simulink model "MotionControlCompile"  (R2016a)
settings: Solver=ode3  StartTime=0.0  StopTime=inf  FixedStep=0.05  RelTol=1e-3
undefined symbols (not defined in the file or in its folder): C_nuParams, D, D_nuParams, InitialPos, invM, invT, invThrustAloc, K2, K3, K4, Kd, Ki, Kp, MAPP1, MAPP2, MAPP3, Sat1Low, Sat1Up, Sat2Low, Sat2Up, Th1, Th2, Th3, Tr, wni, wniCeta2, wnisquared, X, Y, Z
libraries: robotlib x15, marine_gnc x1
settings Model: Creator=einar  LastModifiedBy=einar
settings DataIOCC: LimitDataPoints=on  ReturnWorkspaceOutputs=on
settings OptimizationCC: OptimizeModelRefInitCode=on  LifeSpan=Inf  MaxStackSize=64
settings DebuggingCC: ReadBeforeWriteMsg=DisableAll  WriteAfterWriteMsg=DisableAll  WriteAfterReadMsg=DisableAll  MultiTaskDSMMsg=none  AllowSymbolicDim=off
settings HardwareCC: ProdBitPerPointer=32  ProdLargestAtomicFloat=None  ProdIntDivRoundTo=Undefined  ProdEndianess=Unspecified  ProdWordSize=32  ProdHWDeviceType=Generic->Unspecified (assume 32-bit Generic)
settings ModelReferenceCC: UpdateModelReferenceTargets=IfOutOfDate  PropagateSignalLabelsOutOfModel=off
settings SFSimCC: SFSimEcho=off
settings RTWCC: SystemTargetFile=ert.tlc  HardwareBoard=Robot Operating System (ROS)  TemplateMakefile=ert_default_tmf  Toolchain=Catkin  TargetLang=C++
settings CodeAppCC: IgnoreCustomStorageClasses=off
settings ERTTargetCC: SupportContinuousTime=on  ConvertIfToSwitch=off  SuppressUnreachableDefaultCases=off

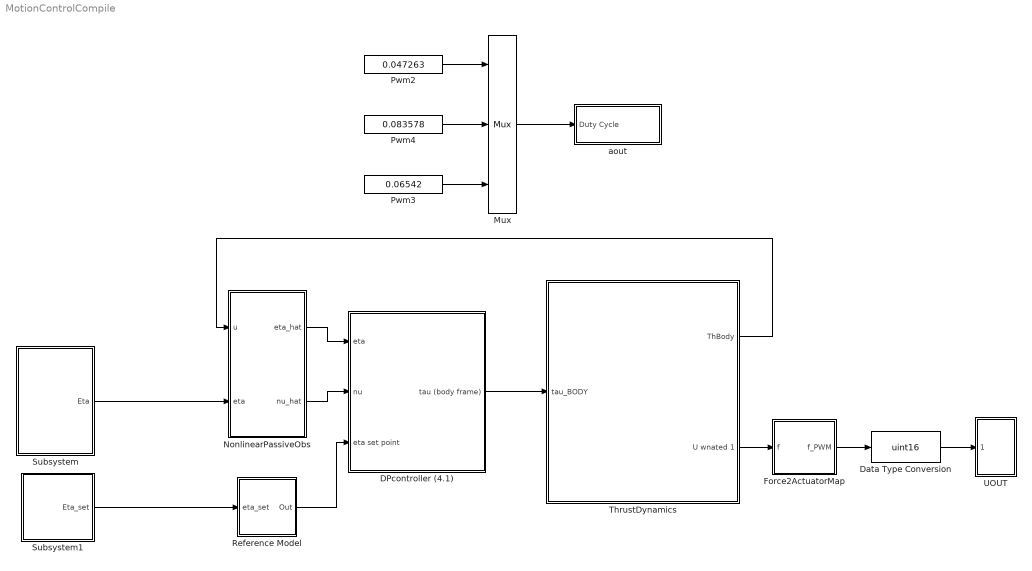
== system MotionControlCompile ==
  DPcontroller (4.1) : Subsystem
  Data Type Conversion : DataTypeConversion  OutDataTypeStr=uint16
  Force2ActuatorMap : Subsystem
  Mux : Mux  Inputs=3
  NonlinearPassiveObs : Subsystem
  Pwm2 : Constant  Value=0.047263
  Pwm3 : Constant  Value=0.06542
  Pwm4 : Constant  Value=0.083578
  Reference Model : Subsystem
  Subsystem : Subsystem
  Subsystem1 : Subsystem
  ThrustDynamics : Subsystem
  UOUT : Subsystem
  aout : Subsystem
  wires:
  NonlinearPassiveObs/2(nu_hat) -> DPcontroller (4.1)/2(nu)
  Reference Model/1(Out) -> DPcontroller (4.1)/3(eta set point)
  NonlinearPassiveObs/1(eta_hat) -> DPcontroller (4.1)/1(eta)
  ThrustDynamics/2(U wnated 1) -> Force2ActuatorMap/1(f)
  Data Type Conversion/1 -> UOUT/1(f_PWM)
  Force2ActuatorMap/1(f_PWM) -> Data Type Conversion/1
  DPcontroller (4.1)/1(tau (body frame)) -> ThrustDynamics/1(tau_BODY)
  ThrustDynamics/1("ThBody ") -> NonlinearPassiveObs/1(u)
  Pwm4/1 -> Mux/2
  Pwm2/1 -> Mux/1
  Pwm3/1 -> Mux/3
  Mux/1 -> aout/1(Duty Cycle)
  Subsystem1/1(Eta_set) -> Reference Model/1(eta_set)
  Subsystem/1(Eta) -> NonlinearPassiveObs/2(eta)

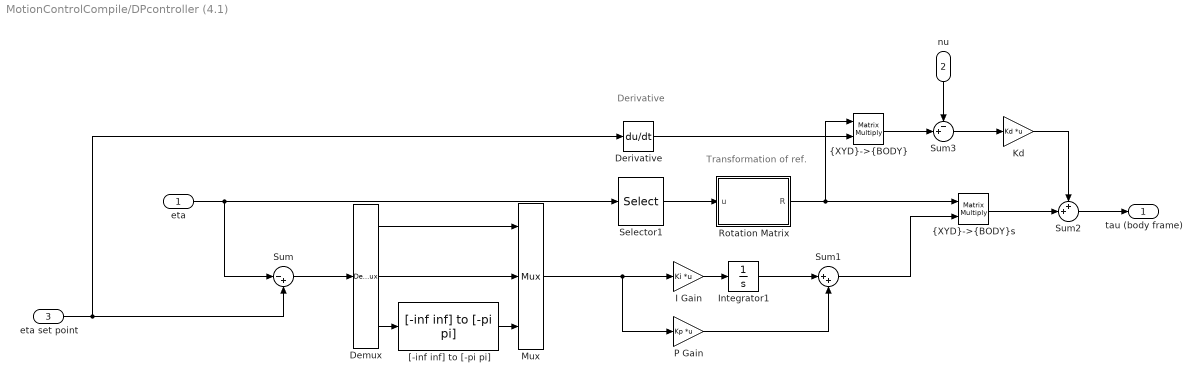
== system MotionControlCompile/DPcontroller (4.1) ==
  note: Transformation of ref.
  note: Derivative
  eta : Inport
  nu : Inport  Port=2
  eta set point : Inport  Port=3
  Demux : Demux  Outputs=3
  Derivative : Derivative
  I Gain : Gain  Gain=Ki  Multiplication=Matrix(K*u)
  Integrator1 : Integrator  InitialCondition=[0;0;0]  LimitOutput=on  UpperSaturationLimit=[1;1;1]  LowerSaturationLimit=[-1;-1;-1]
  Kd : Gain  Gain=Kd  Multiplication=Matrix(K*u)
  Mux : Mux  Inputs=3
  P Gain : Gain  Gain=Kp  Multiplication=Matrix(K*u)
  Rotation Matrix : MATLAB Function  TreatAsAtomicUnit=on
  Selector1 : Selector  InputPortWidth=3  IndexOptions=Index vector (dialog)  Indices=[3]  OutputSizes=1
  Sum : Sum  Inputs=|-+
  Sum1 : Sum  Inputs=|++
  Sum2 : Sum  Inputs=++|
  Sum3 : Sum  Inputs=-+|
  "[-inf inf] to [-pi pi]" : marine_gnc/Utilities/Math Operations/[-inf inf] to [-pi pi]
  "{XYD}->{BODY}" : Product  Multiplication=Matrix(*)
  "{XYD}->{BODY}s" : Product  Multiplication=Matrix(*)
  tau (body frame) : Outport
  wires:
  eta/1 -> Selector1/1, Sum/1
  Selector1/1 -> Rotation Matrix/1(u)
  Rotation Matrix/1(R) -> "{XYD}->{BODY}"/1, "{XYD}->{BODY}s"/1
  Sum2/1 -> tau (body frame)/1
  I Gain/1 -> Integrator1/1
  P Gain/1 -> Sum1/2
  Sum1/1 -> "{XYD}->{BODY}s"/2
  Derivative/1 -> "{XYD}->{BODY}"/2
  "{XYD}->{BODY}s"/1 -> Sum2/2
  nu/1 -> Sum3/1
  "{XYD}->{BODY}"/1 -> Sum3/2
  Sum3/1 -> Kd/1
  Kd/1 -> Sum2/1
  eta set point/1 -> Sum/2, Derivative/1
  Integrator1/1 -> Sum1/1
  Demux/1 -> Mux/1
  Demux/3 -> "[-inf inf] to [-pi pi]"/1
  "[-inf inf] to [-pi pi]"/1 -> Mux/3
  Demux/2 -> Mux/2
  Sum/1 -> Demux/1
  Mux/1 -> P Gain/1, I Gain/1

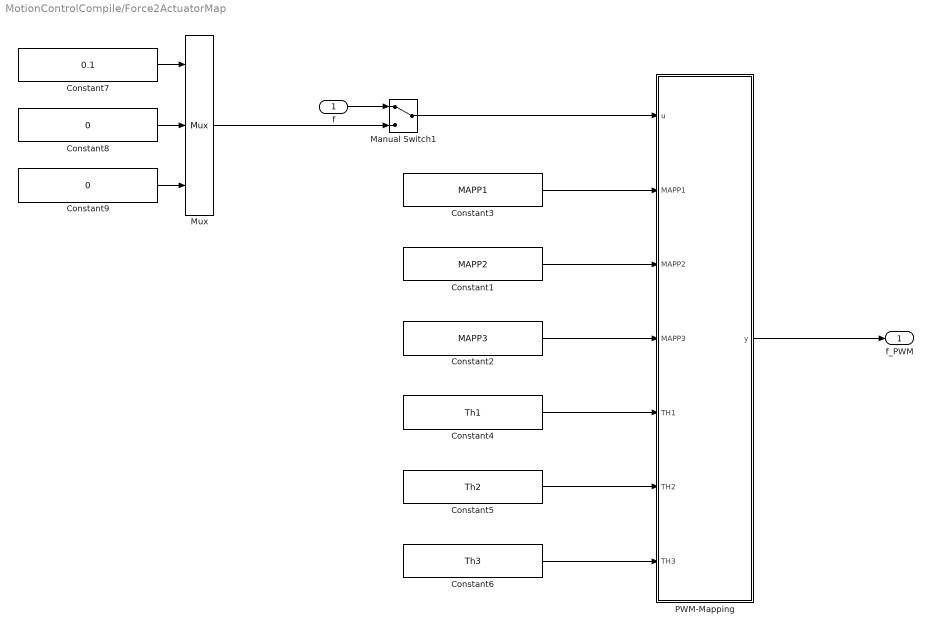
== system MotionControlCompile/Force2ActuatorMap ==
  f : Inport
  Constant1 : Constant  Value=MAPP2
  Constant2 : Constant  Value=MAPP3
  Constant3 : Constant  Value=MAPP1
  Constant4 : Constant  Value=Th1
  Constant5 : Constant  Value=Th2
  Constant6 : Constant  Value=Th3
  Constant7 : Constant  Value=0.1
  Constant8 : Constant  Value=0
  Constant9 : Constant  Value=0
  Manual Switch1 : ManualSwitch
  Mux : Mux  Inputs=3
  PWM-Mapping : MATLAB Function  TreatAsAtomicUnit=on
  f_PWM : Outport
  wires:
  Manual Switch1/1 -> PWM-Mapping/1(u)
  Constant4/1 -> PWM-Mapping/5(TH1)
  Constant6/1 -> PWM-Mapping/7(TH3)
  Constant5/1 -> PWM-Mapping/6(TH2)
  Constant3/1 -> PWM-Mapping/2(MAPP1)
  Constant1/1 -> PWM-Mapping/3(MAPP2)
  Constant2/1 -> PWM-Mapping/4(MAPP3)
  PWM-Mapping/1(y) -> f_PWM/1
  f/1 -> Manual Switch1/1
  Constant7/1 -> Mux/1
  Constant8/1 -> Mux/2
  Mux/1 -> Manual Switch1/2
  Constant9/1 -> Mux/3

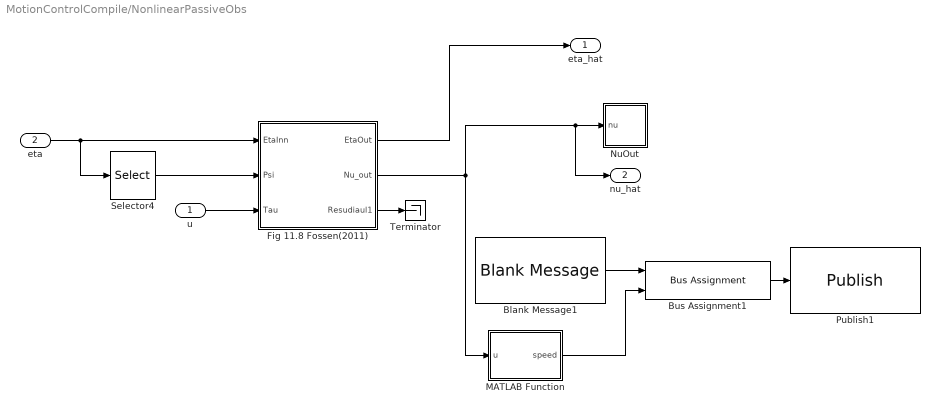
== system MotionControlCompile/NonlinearPassiveObs ==
  u : Inport
  eta : Inport  Port=2
  Blank Message1 : robotlib/Blank Message  SourceLibraryInfo=This block requires Robotics System Toolbox  messageType=std_msgs/Float64  SampleTime=inf
  Bus Assignment1 : BusAssignment  AssignedSignals=Data
  Fig 11.8 Fossen(2011) : Subsystem
  MATLAB Function : MATLAB Function  TreatAsAtomicUnit=on
  NuOut : Subsystem
  Publish1 : robotlib/Publish  SourceLibraryInfo=This block requires Robotics System Toolbox  topicSource=Specify your own  topic=/VesselSpeed  messageType=std_msgs/Float64  messageQueueLength=1
  Selector4 : Selector  InputPortWidth=3  IndexOptions=Index vector (dialog)  Indices=3  OutputSizes=1
  Terminator : Terminator
  eta_hat : Outport
  nu_hat : Outport  Port=2
  wires:
  Fig 11.8 Fossen(2011)/3("Resudiaul1 ") -> Terminator/1
  eta/1 -> Fig 11.8 Fossen(2011)/1(EtaInn), Selector4/1
  Selector4/1 -> Fig 11.8 Fossen(2011)/2(Psi)
  u/1 -> Fig 11.8 Fossen(2011)/3("Tau ")
  Fig 11.8 Fossen(2011)/1("EtaOut ") -> eta_hat/1
  Bus Assignment1/1 -> Publish1/1
  Blank Message1/1 -> Bus Assignment1/1
  Fig 11.8 Fossen(2011)/2("Nu_out ") -> nu_hat/1, NuOut/1("nu "), MATLAB Function/1(u)
  MATLAB Function/1(speed) -> Bus Assignment1/2

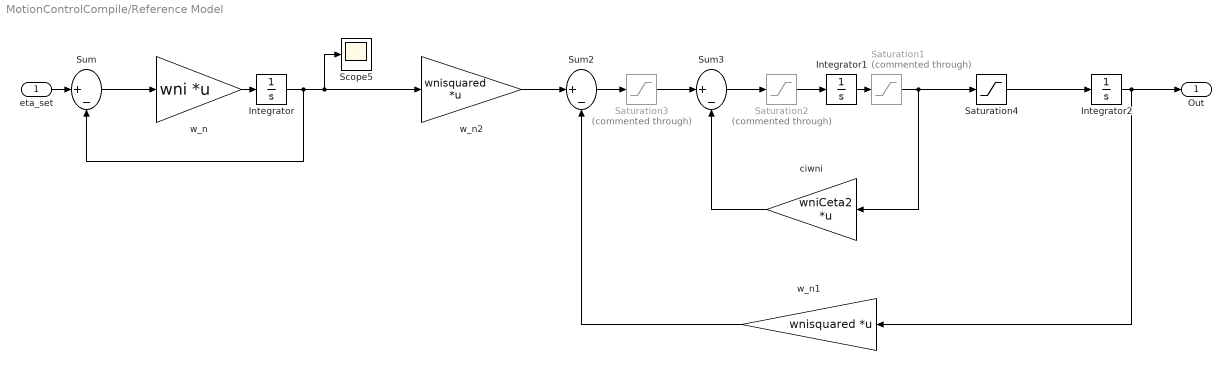
== system MotionControlCompile/Reference Model ==
  eta_set : Inport
  Integrator : Integrator  InitialCondition=[0;0;0]
  Integrator1 : Integrator  InitialCondition=[0 ;0; 0]
  Integrator2 : Integrator  InitialCondition=[0;0;0]
  Saturation1 : Saturate  Commented=through  UpperLimit=Sat2Up  LowerLimit=Sat2Low
  Saturation2 : Saturate  Commented=through  UpperLimit=Sat1Up  LowerLimit=Sat1Low
  Saturation3 : Saturate  Commented=through  UpperLimit=Sat1Up  LowerLimit=Sat1Low
  Saturation4 : Saturate  UpperLimit=Sat2Up  LowerLimit=Sat2Low
  Scope5 : Scope
  Sum : Sum  Inputs=|+-
  Sum2 : Sum  Inputs=|+-
  Sum3 : Sum  Inputs=|+-
  ciwni : Gain  Gain=wniCeta2  Multiplication=Matrix(K*u)
  w_n : Gain  Gain=wni  Multiplication=Matrix(K*u)
  w_n1 : Gain  Gain=wnisquared  Multiplication=Matrix(K*u)
  w_n2 : Gain  Gain=wnisquared  Multiplication=Matrix(K*u)
  Out : Outport
  wires:
  w_n/1 -> Integrator/1
  w_n2/1 -> Sum2/1
  Integrator/1 -> Scope5/1, w_n2/1, Sum/2
  Integrator2/1 -> Out/1, w_n1/1
  ciwni/1 -> Sum3/2
  Saturation1/1 -> ciwni/1, Saturation4/1
  Saturation2/1 -> Integrator1/1
  Sum2/1 -> Saturation3/1
  Sum3/1 -> Saturation2/1
  Sum/1 -> w_n/1
  eta_set/1 -> Sum/1
  Integrator1/1 -> Saturation1/1
  w_n1/1 -> Sum2/2
  Saturation3/1 -> Sum3/1
  Saturation4/1 -> Integrator2/1

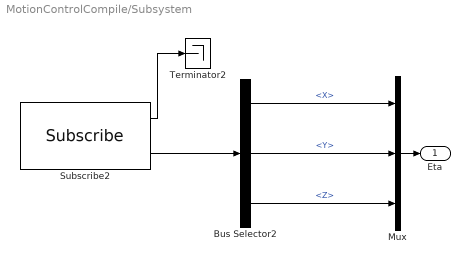
== system MotionControlCompile/Subsystem ==
  Bus Selector2 : BusSelector  OutputSignals=X,Y,Z
  Mux : Mux  Inputs=3
  Subscribe2 : robotlib/Subscribe  SourceLibraryInfo=This block requires Robotics System Toolbox  topicSource=Specify your own  topic=/Position  messageType=geometry_msgs/Vector3  sampleTime=-1  messageQueueLength=1
  Terminator2 : Terminator
  Eta : Outport
  wires:
  Bus Selector2/1 -> Mux/1  "<X>"
  Subscribe2/2 -> Bus Selector2/1
  Mux/1 -> Eta/1
  Subscribe2/1 -> Terminator2/1
  Bus Selector2/3 -> Mux/3  "<Z>"
  Bus Selector2/2 -> Mux/2  "<Y>"

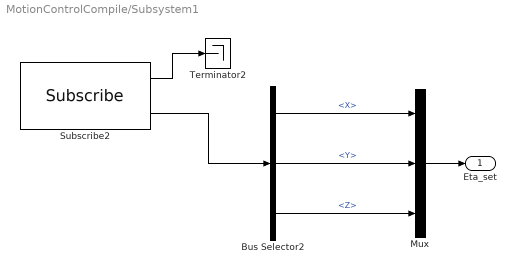
== system MotionControlCompile/Subsystem1 ==
  Bus Selector2 : BusSelector  OutputSignals=X,Y,Z
  Mux : Mux  Inputs=3
  Subscribe2 : robotlib/Subscribe  SourceLibraryInfo=This block requires Robotics System Toolbox  topicSource=Specify your own  topic=/SetPoint  messageType=geometry_msgs/Vector3  sampleTime=-1  messageQueueLength=1
  Terminator2 : Terminator
  Eta_set : Outport
  wires:
  Subscribe2/2 -> Bus Selector2/1
  Mux/1 -> Eta_set/1
  Subscribe2/1 -> Terminator2/1
  Bus Selector2/1 -> Mux/1  "<X>"
  Bus Selector2/2 -> Mux/2  "<Y>"
  Bus Selector2/3 -> Mux/3  "<Z>"

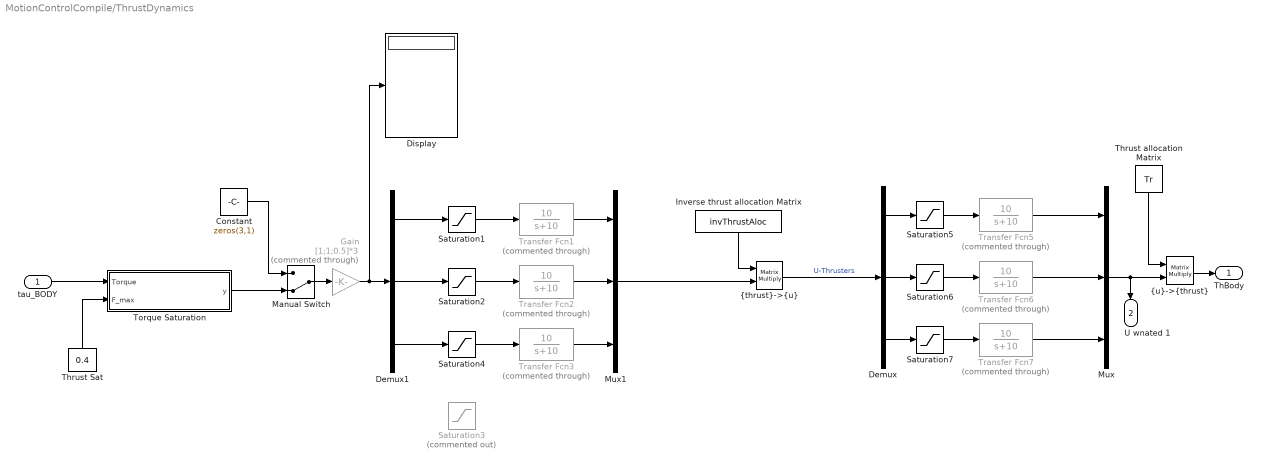
== system MotionControlCompile/ThrustDynamics ==
  tau_BODY : Inport
  Constant : Constant  Value=zeros(3,1)
  Demux : Demux  Outputs=3
  Demux1 : Demux  Outputs=3
  Display : Display
  Gain : Gain  Commented=through  Gain=[1;1;0.5]*3
  Inverse thrust allocation Matrix : Constant  Value=invThrustAloc
  Manual Switch : ManualSwitch  CurrentSetting=0
  Mux : Mux  Inputs=3
  Mux1 : Mux  Inputs=3
  Saturation1 : Saturate  UpperLimit=1  LowerLimit=-1  ZeroCross=off
  Saturation2 : Saturate  UpperLimit=1  LowerLimit=-1  ZeroCross=off
  Saturation3 : Saturate  Commented=on  UpperLimit=0.05  LowerLimit=-0.05  ZeroCross=off
  Saturation4 : Saturate  UpperLimit=1  LowerLimit=-1  ZeroCross=off
  Saturation5 : Saturate  UpperLimit=4  LowerLimit=-4  ZeroCross=off
  Saturation6 : Saturate  UpperLimit=4  LowerLimit=-4  ZeroCross=off
  Saturation7 : Saturate  UpperLimit=4  LowerLimit=-4  ZeroCross=off
  Thrust Sat : Constant  Value=0.4
  Thrust allocation Matrix : Constant  Value=Tr
  Torque Saturation : MATLAB Function  TreatAsAtomicUnit=on
  Transfer Fcn{1..3,5..7} (6 alike) : TransferFcn  Commented=through  Numerator=[10]  Denominator=[1 10]
  "{thrust}->{u}" : Product  Multiplication=Matrix(*)
  "{u}->{thrust}" : Product  Multiplication=Matrix(*)
  "ThBody " : Outport
  U wnated 1 : Outport  Port=2
  wires:
  Demux/1 -> Saturation5/1
  Demux/2 -> Saturation6/1
  Demux/3 -> Saturation7/1
  "{u}->{thrust}"/1 -> "ThBody "/1
  Thrust allocation Matrix/1 -> "{u}->{thrust}"/1
  Mux/1 -> "{u}->{thrust}"/2, U wnated 1/1
  "{thrust}->{u}"/1 -> Demux/1  "U-Thrusters"
  Inverse thrust allocation Matrix/1 -> "{thrust}->{u}"/1
  Saturation7/1 -> Transfer Fcn7/1
  Saturation6/1 -> Transfer Fcn6/1
  Saturation5/1 -> Transfer Fcn5/1
  Transfer Fcn5/1 -> Mux/1
  Transfer Fcn7/1 -> Mux/3
  Transfer Fcn6/1 -> Mux/2
  tau_BODY/1 -> Torque Saturation/1(Torque)
  Demux1/1 -> Saturation1/1
  Demux1/2 -> Saturation2/1
  Demux1/3 -> Saturation4/1
  Saturation4/1 -> Transfer Fcn3/1
  Saturation2/1 -> Transfer Fcn2/1
  Saturation1/1 -> Transfer Fcn1/1
  Transfer Fcn1/1 -> Mux1/1
  Transfer Fcn3/1 -> Mux1/3
  Transfer Fcn2/1 -> Mux1/2
  Gain/1 -> Display/1, Demux1/1
  Mux1/1 -> "{thrust}->{u}"/2
  Thrust Sat/1 -> Torque Saturation/2(F_max)
  Torque Saturation/1(y) -> Manual Switch/2
  Manual Switch/1 -> Gain/1
  Constant/1 -> Manual Switch/1

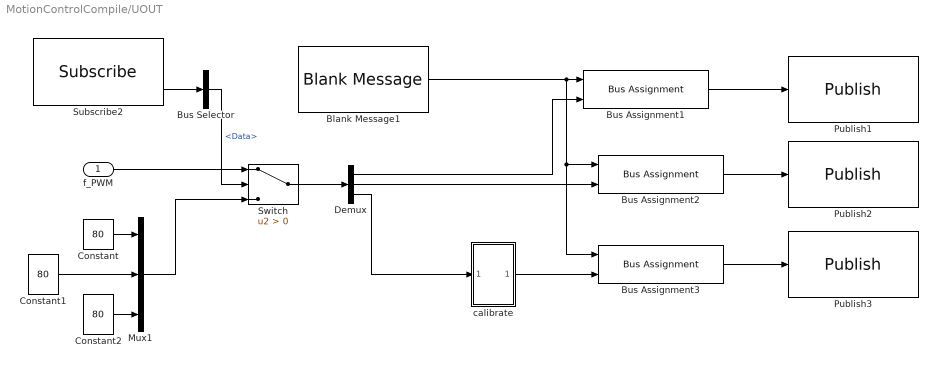
== system MotionControlCompile/UOUT ==
  f_PWM : Inport
  Blank Message1 : robotlib/Blank Message  SourceLibraryInfo=This block requires Robotics System Toolbox  messageType=std_msgs/UInt16  SampleTime=inf
  Bus Assignment1 : BusAssignment  AssignedSignals=Data
  Bus Assignment2 : BusAssignment  AssignedSignals=Data
  Bus Assignment3 : BusAssignment  AssignedSignals=Data
  Bus Selector : BusSelector  OutputSignals=Data
  Constant : Constant  Value=80  OutDataTypeStr=uint16
  Constant1 : Constant  Value=80  OutDataTypeStr=uint16
  Constant2 : Constant  Value=80  OutDataTypeStr=uint16
  Demux : Demux  Outputs=3
  Mux1 : Mux  Inputs=3
  Publish1 : robotlib/Publish  SourceLibraryInfo=This block requires Robotics System Toolbox  topicSource=Specify your own  topic=/Thrust1  messageType=std_msgs/UInt16  messageQueueLength=1
  Publish2 : robotlib/Publish  SourceLibraryInfo=This block requires Robotics System Toolbox  topicSource=Specify your own  topic=/Thrust2  messageType=std_msgs/UInt16  messageQueueLength=1
  Publish3 : robotlib/Publish  SourceLibraryInfo=This block requires Robotics System Toolbox  topicSource=Specify your own  topic=/Thrust3  messageType=std_msgs/UInt16  messageQueueLength=1
  Subscribe2 : robotlib/Subscribe  SourceLibraryInfo=This block requires Robotics System Toolbox  topicSource=Specify your own  topic=/Motor_on_off  messageType=std_msgs/Bool  sampleTime=-1  messageQueueLength=1
  Switch : Switch  Criteria=u2 > Threshold
  calibrate : Subsystem
  wires:
  Bus Assignment3/1 -> Publish3/1
  Demux/2 -> Bus Assignment2/2
  Bus Assignment1/1 -> Publish1/1
  Blank Message1/1 -> Bus Assignment3/1, Bus Assignment2/1, Bus Assignment1/1
  f_PWM/1 -> Switch/1
  Demux/1 -> Bus Assignment1/2
  Bus Assignment2/1 -> Publish2/1
  Switch/1 -> Demux/1
  Mux1/1 -> Switch/3
  Constant/1 -> Mux1/1
  Constant1/1 -> Mux1/2
  Constant2/1 -> Mux1/3
  Subscribe2/2 -> Bus Selector/1
  Bus Selector/1 -> Switch/2  "<Data>"
  Demux/3 -> calibrate/1(In1)
  calibrate/1(Out1) -> Bus Assignment3/2

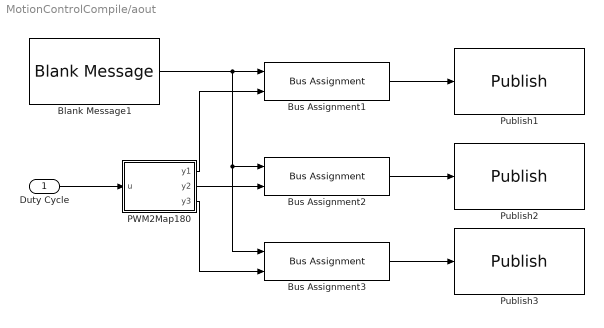
== system MotionControlCompile/aout ==
  Duty Cycle : Inport
  Blank Message1 : robotlib/Blank Message  SourceLibraryInfo=This block requires Robotics System Toolbox  messageType=std_msgs/UInt16  SampleTime=inf
  Bus Assignment1 : BusAssignment  AssignedSignals=Data
  Bus Assignment2 : BusAssignment  AssignedSignals=Data
  Bus Assignment3 : BusAssignment  AssignedSignals=Data
  PWM2Map180 : MATLAB Function  TreatAsAtomicUnit=on
  Publish1 : robotlib/Publish  SourceLibraryInfo=This block requires Robotics System Toolbox  topicSource=Specify your own  topic=/a1  messageType=std_msgs/UInt16  messageQueueLength=1
  Publish2 : robotlib/Publish  SourceLibraryInfo=This block requires Robotics System Toolbox  topicSource=Specify your own  topic=/a2  messageType=std_msgs/UInt16  messageQueueLength=1
  Publish3 : robotlib/Publish  SourceLibraryInfo=This block requires Robotics System Toolbox  topicSource=Specify your own  topic=/a3  messageType=std_msgs/UInt16  messageQueueLength=1
  wires:
  Bus Assignment2/1 -> Publish2/1
  PWM2Map180/1(y1) -> Bus Assignment1/2
  PWM2Map180/3(y3) -> Bus Assignment3/2
  Duty Cycle/1 -> PWM2Map180/1(u)
  Blank Message1/1 -> Bus Assignment1/1, Bus Assignment2/1, Bus Assignment3/1
  Bus Assignment1/1 -> Publish1/1
  PWM2Map180/2(y2) -> Bus Assignment2/2
  Bus Assignment3/1 -> Publish3/1

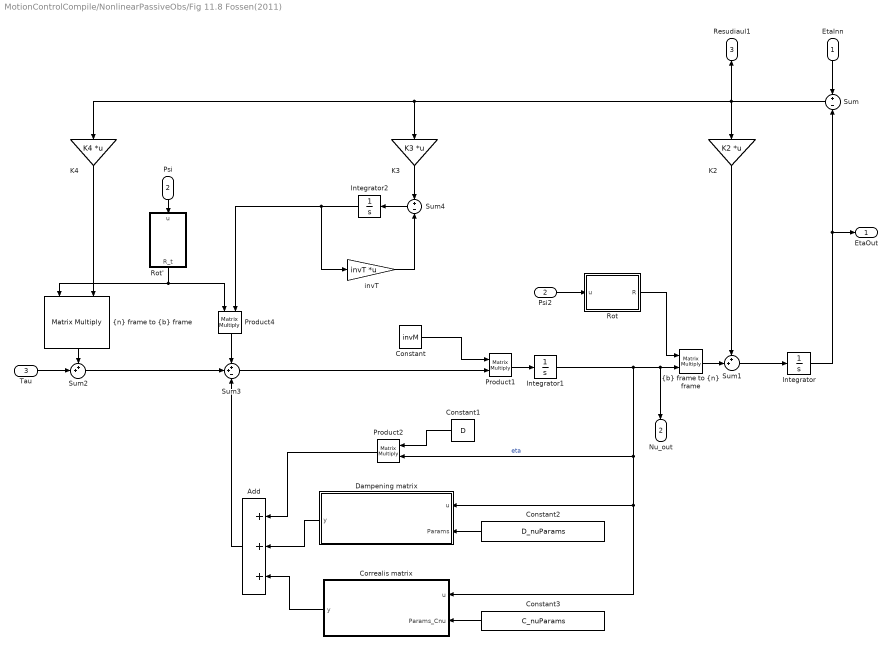
== system MotionControlCompile/NonlinearPassiveObs/Fig 11.8 Fossen(2011) ==
  EtaInn : Inport
  Psi : Inport  Port=2
  "Tau " : Inport  Port=3
  Add : Sum  Inputs=+++
  Constant : Constant  Value=invM
  Constant1 : Constant  Value=D
  Constant2 : Constant  Value=D_nuParams
  Constant3 : Constant  Value=C_nuParams
  Correalis matrix : MATLAB Function  TreatAsAtomicUnit=on
  Dampening matrix : MATLAB Function  TreatAsAtomicUnit=on
  Integrator : Integrator  InitialCondition=InitialPos
  Integrator1 : Integrator
  Integrator2 : Integrator  InitialCondition=[0;0;0]
  K2 : Gain  Gain=K2  Multiplication=Matrix(K*u)
  K3 : Gain  Gain=K3  Multiplication=Matrix(K*u)
  K4 : Gain  Gain=K4  Multiplication=Matrix(K*u)
  Product1 : Product  Multiplication=Matrix(*)
  Product2 : Product  Multiplication=Matrix(*)
  Product4 : Product  Multiplication=Matrix(*)
  Psi2 : InportShadow  Port=2
  Rot : MATLAB Function  TreatAsAtomicUnit=on
  Rot' : MATLAB Function  TreatAsAtomicUnit=on
  Sum : Sum  Inputs=+|-
  Sum1 : Sum  Inputs=++|
  Sum2 : Sum  Inputs=++|
  Sum3 : Sum  Inputs=++-
  Sum4 : Sum  Inputs=+|-
  invT : Gain  Gain=invT  Multiplication=Matrix(K*u)
  "{b} frame to {n} frame" : Product  Multiplication=Matrix(*)
  "{n} frame to {b} frame" : Product  Multiplication=Matrix(*)
  "EtaOut " : Outport
  "Nu_out " : Outport  Port=2
  "Resudiaul1 " : Outport  Port=3
  wires:
  Add/1 -> Sum3/3
  Correalis matrix/1(y) -> Add/3
  Dampening matrix/1(y) -> Add/2
  Product2/1 -> Add/1
  Integrator1/1 -> "{b} frame to {n} frame"/2, "Nu_out "/1, Product2/2, Dampening matrix/1(u), Correalis matrix/1(u)  "eta"
  Constant3/1 -> Correalis matrix/2(Params_Cnu)
  Constant2/1 -> Dampening matrix/2(Params)
  K4/1 -> "{n} frame to {b} frame"/2
  EtaInn/1 -> Sum/1
  Sum/1 -> "Resudiaul1 "/1, K4/1, K3/1, K2/1
  K2/1 -> Sum1/1
  Sum1/1 -> Integrator/1
  Integrator/1 -> Sum/2, "EtaOut "/1
  Psi/1 -> Rot'/1(u)
  "{n} frame to {b} frame"/1 -> Sum2/1
  "Tau "/1 -> Sum2/2
  Constant/1 -> Product1/1
  Product1/1 -> Integrator1/1
  Constant1/1 -> Product2/1
  Sum2/1 -> Sum3/2
  Sum3/1 -> Product1/2
  Psi2/1 -> Rot/1(u)
  Rot/1(R) -> "{b} frame to {n} frame"/1
  Rot'/1(R_t) -> "{n} frame to {b} frame"/1, Product4/1
  "{b} frame to {n} frame"/1 -> Sum1/2
  K3/1 -> Sum4/1
  Sum4/1 -> Integrator2/1
  Integrator2/1 -> Product4/2, invT/1
  invT/1 -> Sum4/2
  Product4/1 -> Sum3/1

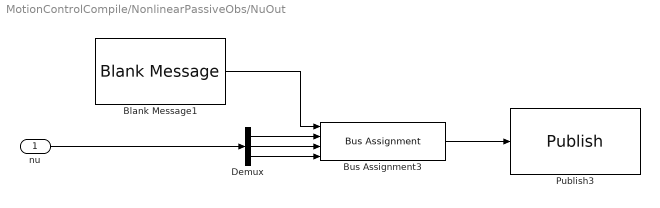
== system MotionControlCompile/NonlinearPassiveObs/NuOut ==
  "nu " : Inport
  Blank Message1 : robotlib/Blank Message  SourceLibraryInfo=This block requires Robotics System Toolbox  messageType=geometry_msgs/Vector3  SampleTime=inf
  Bus Assignment3 : BusAssignment  AssignedSignals=X,Y,Z
  Demux : Demux  Outputs=3
  Publish3 : robotlib/Publish  SourceLibraryInfo=This block requires Robotics System Toolbox  topicSource=Specify your own  topic=/nu  messageType=geometry_msgs/Vector3  messageQueueLength=1
  wires:
  Bus Assignment3/1 -> Publish3/1
  Blank Message1/1 -> Bus Assignment3/1
  "nu "/1 -> Demux/1
  Demux/1 -> Bus Assignment3/2
  Demux/2 -> Bus Assignment3/3
  Demux/3 -> Bus Assignment3/4

== system MotionControlCompile/UOUT/calibrate ==
  In1 : Inport
  Calibrate : MATLAB Function  TreatAsAtomicUnit=on
  Data Type Conversion : DataTypeConversion  OutDataTypeStr=int16
  Data Type Conversion1 : DataTypeConversion  OutDataTypeStr=uint16
  Out1 : Outport
  wires:
  Data Type Conversion/1 -> Calibrate/1(u)
  Calibrate/1(y) -> Data Type Conversion1/1
  Data Type Conversion1/1 -> Out1/1
  In1/1 -> Data Type Conversion/1

== matlab function MotionControlCompile/DPcontroller (4.1)/Rotation Matrix ==
  data: u input; R output
function R = fcn(u)
RotPhi=[cos(u) -sin(u) 0;sin(u) cos(u) 0 ;0 0 1];
R = RotPhi';
%R=[RotPhi(1:2,:);[0 0 0;0 0 0;0 0 0];RotPhi(3,:)]
end

== matlab function MotionControlCompile/NonlinearPassiveObs/Fig 11.8 Fossen(2011)/Correalis matrix ==
  data: u input; y output; Params_Cnu input
function y = fcn(u,Params_Cnu)
%#codegen
C=[0 Params_Cnu(2,1)*u(3) 0;-Params_Cnu(1,2)*u(3) 0 0;0 0 0];
y=C*u;

== matlab function MotionControlCompile/NonlinearPassiveObs/Fig 11.8 Fossen(2011)/Dampening matrix ==
  data: u input; y output; Params input
function y = fcn(u,Params)
%#codegen
Dnu=[Params(1,1)*abs(u(1)) 0 0;0 Params(2,2)*abs(u(2)) 0;0 0 0];
y=Dnu*u;

== matlab function MotionControlCompile/Force2ActuatorMap/PWM-Mapping ==
  data: u input; y output; MAPP1 input; MAPP2 input; MAPP3 input; TH1 input; TH2 input; TH3 input
function y = fcn(u,MAPP1,MAPP2,MAPP3,TH1,TH2,TH3)
y=[0 ;0;0]
u(3)=-u(3);
MAPP3=-MAPP1;
TH3=TH1

if u(1)>max(MAPP1)
    u(1)=max(MAPP1)
elseif u(1)<min(MAPP1)
u(1)=min(MAPP1);
end

if u(2)>max(MAPP2)
    u(2)=max(MAPP2)
elseif u(2)<min(MAPP2)
u(2)=min(MAPP2);
end

if u(3)>max(MAPP3)
    u(3)=max(MAPP3)
elseif u(3)<min(MAPP3)
u(3)=min(MAPP3);
end

y(1)=interp1(MAPP1,TH1,u(1))
y(2)=interp1(MAPP2,TH2,u(2))
y(3)=interp1(MAPP3,TH3,u(3))

if abs(u(1))<0.01
    y(1)=80;
end
if abs(u(2))<0.01
    y(2)=80;
end
if abs(u(3))<0.01
    y(3)=80;
end

== matlab function MotionControlCompile/UOUT/calibrate/Calibrate ==
  data: u input; y output
function y  = fcn(u)
y=u;
if u<80
y=y+3
end
%     y=y+1;
% elseif u<80
%     y=y+3;
% end

== matlab function MotionControlCompile/NonlinearPassiveObs/Fig 11.8 Fossen(2011)/Rot' ==
  data: u input; R_t output
function R_t = fcn(u)
RotPhi=[cos(u) -sin(u) 0;sin(u) cos(u) 0 ;0 0 1];
R_t = RotPhi';
%R=[RotPhi(1:2,:);[0 0 0;0 0 0;0 0 0];RotPhi(3,:)]
end

== matlab function MotionControlCompile/NonlinearPassiveObs/MATLAB Function ==
  data: u input; speed output
function speed = fcn(u)
%#codegen
speed=norm(u(1:2));

== matlab function MotionControlCompile/NonlinearPassiveObs/Fig 11.8 Fossen(2011)/Rot ==
  data: u input; R output
function R = fcn(u)
RotPhi=[cos(u) -sin(u) 0;sin(u) cos(u) 0 ;0 0 1];
R = RotPhi;
end

== matlab function MotionControlCompile/ThrustDynamics/Torque Saturation ==
  data: Torque input; y output; F_max input
function y = fcn(Torque,F_max)
Com_Torque=norm(Torque(1:2));
if Com_Torque>F_max
    Torque(1:2,1)=Torque(1:2,1).*(F_max/Com_Torque);
end
T_max=0.3;
if abs(Torque(3))>T_max
    Torque(3)=T_max*Torque(3)/abs(Torque(3));
end;
y=Torque;

== matlab function MotionControlCompile/aout/PWM2Map180 ==
  data: u input; y1 output; y2 output; y3 output
function [y1,y2,y3] = fcn(u)
%#codegen
y1=uint16((u(1)-0.027)*180/0.093);
y2=uint16((u(2)-0.027)*180/0.093);
y3=uint16((u(3)-0.027)*180/0.093);
